simulink model "powerwindow05"  (Simulink 6.0)
settings: Solver=ode23t  StartTime=0.0  StopTime=inf  FixedStep=1e-4  RelTol=1e-2
InitFcn:
  | powericon('psbinitsys',bdroot);
values from neighbouring files (symbols this model uses):
  m = 50    [absdata.m]
libraries: powerlib x44, mblibv1 x18, simulink x8, dspquant2 x5, xpclib x4
(part 1 of 2)
settings Model: Creator=The MathWorks Inc.  LastModifiedBy=batserve  ExtModeAutoUpdateStatusClock=off
settings DataIOCC: SignalLoggingName=sigsOut
settings OptimizationCC: BooleanDataType=off
settings DebuggingCC: CheckExecutionContextPreStartOutputMsg=on  CheckExecutionContextRuntimeOutputMsg=on  SolverPrmCheckMsg=none  ParameterPrecisionLossMsg=none
settings HardwareCC: TargetUnknown=on
settings SimMechanicsCC: VisOnUpdateDiagram=on

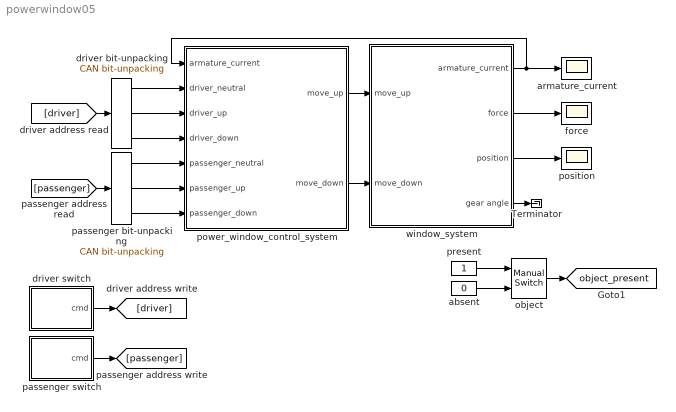
== system powerwindow05 ==
  Terminator : Terminator
  absent : Constant  Value=0
  armature_current : Scope
      settings: DataFormat=Array
  driver bit-unpacking : xpclib/CAN/Utilities/CAN bit-unpacking   bitpatterns={ [0:0] [1:1] [2:2] }  dtypes={ 'boolean' 'boolean' 'boolean' }
  driver switch : Subsystem  PropExecContextAcrossSSBoundary=on
  force : Scope
      settings: DataFormat=Array
  object : simulink/Signal Routing/Manual Switch  sw=1  action=0
  passenger bit-unpacking : xpclib/CAN/Utilities/CAN bit-unpacking   bitpatterns={ [0:0] [1:1] [2:2] }  dtypes={ 'boolean' 'boolean' 'boolean' }
  passenger switch : Subsystem  PropExecContextAcrossSSBoundary=on
  position : Scope
      settings: YMin=-0.05  YMax=0.5  DataFormat=Array
  power_window_control_system : Subsystem  PropExecContextAcrossSSBoundary=on
  present : Constant
  window_system : Subsystem  AncestorBlock=powerwindowlibphys/detailed_window_system  PropExecContextAcrossSSBoundary=on
  tag scope: object_present=global
  wires:
  power_window_control_system/1(move_up) -> window_system/1(move_up)
  power_window_control_system/2(move_down) -> window_system/2(move_down)
  window_system/1(armature_current) -> armature_current/1, power_window_control_system/1(armature_current)
  window_system/2(force) -> force/1
  window_system/3(position) -> position/1
  present/1 -> object/1
  absent/1 -> object/2
  object/1 -> [object_present]
  [passenger] -> passenger bit-unpacking/1
  [driver] -> driver bit-unpacking/1
  driver bit-unpacking/1 -> power_window_control_system/2(driver_neutral)
  driver bit-unpacking/2 -> power_window_control_system/3(driver_up)
  driver bit-unpacking/3 -> power_window_control_system/4(driver_down)
  passenger bit-unpacking/1 -> power_window_control_system/5(passenger_neutral)
  passenger bit-unpacking/2 -> power_window_control_system/6(passenger_up)
  passenger bit-unpacking/3 -> power_window_control_system/7(passenger_down)
  passenger switch/1(cmd) -> [passenger]
  driver switch/1(cmd) -> [driver]
  window_system/4(gear angle) -> Terminator/1

== system powerwindow05/driver switch ==
  CAN module : Subsystem  PropExecContextAcrossSSBoundary=on
  DAQ : Subsystem  PropExecContextAcrossSSBoundary=on
  GND : powerlib/Elements/Ground  Orientation=down  PhysicalDomain=powersysdomain  SubClassName=unknown  LeftPortType=p1  RightPortType=p1  LConnTagsString=a
  Vbattery 12[V] : powerlib/Electrical Sources/DC Voltage Source  Amplitude=12  Measurements=None
  control : Subsystem  PropExecContextAcrossSSBoundary=on
  switch : Subsystem  PropExecContextAcrossSSBoundary=on
  cmd : Outport
  wires:
  control/1(cmd) -> CAN module/1(command)
  CAN module/1(3bit) -> cmd/1
  DAQ/1(Out1) -> control/1(up)
  DAQ/2(Out2) -> control/2(down)
  connections:
  switch/RConn1 -- DAQ/LConn1
  switch/RConn2 -- DAQ/LConn2
  GND/LConn1 -- Vbattery 12[V]/LConn1
  Vbattery 12[V]/RConn1 -- switch/LConn1

== system powerwindow05/passenger switch ==
  CAN module : Subsystem  PropExecContextAcrossSSBoundary=on
  DAQ : Subsystem  PropExecContextAcrossSSBoundary=on
  GND : powerlib/Elements/Ground  Orientation=down  PhysicalDomain=powersysdomain  SubClassName=unknown  LeftPortType=p1  RightPortType=p1  LConnTagsString=a
  Vbattery 12[V] : powerlib/Electrical Sources/DC Voltage Source  Amplitude=12  Measurements=None
  control : Subsystem  PropExecContextAcrossSSBoundary=on
  switch : Subsystem  PropExecContextAcrossSSBoundary=on
  cmd : Outport
  wires:
  DAQ/2(Out2) -> control/2(down)
  DAQ/1(Out1) -> control/1(up)
  CAN module/1(3bit) -> cmd/1
  control/1(cmd) -> CAN module/1(command)
  connections:
  Vbattery 12[V]/RConn1 -- switch/LConn1
  GND/LConn1 -- Vbattery 12[V]/LConn1
  switch/RConn2 -- DAQ/LConn2
  switch/RConn1 -- DAQ/LConn1

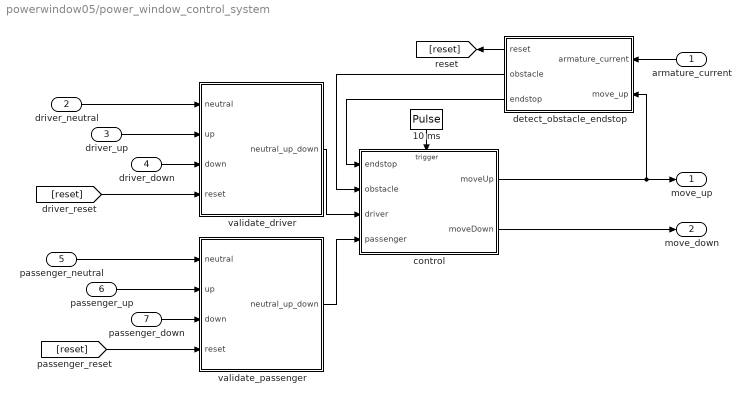
== system powerwindow05/power_window_control_system ==
  armature_current : Inport  Orientation=left  Port=1  LatchInput=off
  driver_neutral : Inport  Port=2  LatchInput=off
  driver_up : Inport  Port=3  LatchInput=off
  driver_down : Inport  Port=4  LatchInput=off
  passenger_neutral : Inport  Port=5  LatchInput=off
  passenger_up : Inport  Port=6  LatchInput=off
  passenger_down : Inport  Port=7  LatchInput=off
  10 ms : DiscretePulseGenerator  Orientation=down  SampleTime=10e-3
  control : Stateflow chart  TreatAsAtomicUnit=on  PropExecContextAcrossSSBoundary=on
  detect_obstacle_endstop : Subsystem  Orientation=left  PropExecContextAcrossSSBoundary=on
  validate_driver : Subsystem  PropExecContextAcrossSSBoundary=on
  validate_passenger : Subsystem  PropExecContextAcrossSSBoundary=on
  move_up : Outport
  move_down : Outport  Port=2
  wires:
  detect_obstacle_endstop/2(obstacle) -> control/2(obstacle)
  detect_obstacle_endstop/3(endstop) -> control/1(endstop)
  detect_obstacle_endstop/1(reset) -> [reset]
  armature_current/1 -> detect_obstacle_endstop/1(armature_current)
  10 ms/1 -> control/Trigger
  control/1(moveUp) -> detect_obstacle_endstop/2(move_up), move_up/1
  control/2(moveDown) -> move_down/1
  driver_neutral/1 -> validate_driver/1(neutral)
  driver_up/1 -> validate_driver/2(up)
  driver_down/1 -> validate_driver/3(down)
  [reset] -> validate_driver/4(reset)
  passenger_neutral/1 -> validate_passenger/1(neutral)
  passenger_up/1 -> validate_passenger/2(up)
  passenger_down/1 -> validate_passenger/3(down)
  [reset] -> validate_passenger/4(reset)
  validate_driver/1(neutral_up_down) -> control/3(driver)
  validate_passenger/1(neutral_up_down) -> control/4(passenger)

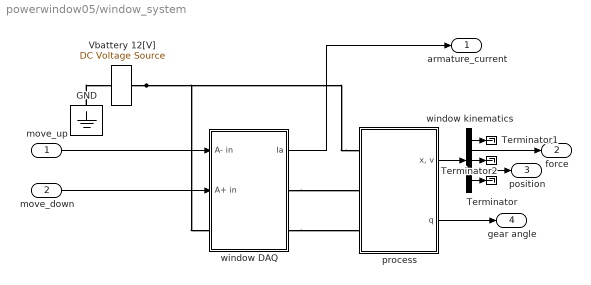
== system powerwindow05/window_system ==
  move_up : Inport  Port=1  LatchInput=off
  move_down : Inport  Port=2  LatchInput=off
  GND : powerlib/Elements/Ground  Orientation=down  PhysicalDomain=powersysdomain  SubClassName=unknown  LeftPortType=p1  RightPortType=p1  LConnTagsString=a
  Terminator : Terminator
  Terminator1 : Terminator
  Terminator2 : Terminator
  Vbattery 12[V] : powerlib/Electrical Sources/DC Voltage Source  Amplitude=12  Measurements=None
  process : Subsystem  AncestorBlock=powerwindowlibphys/process  PropExecContextAcrossSSBoundary=on
  window DAQ : Subsystem  PropExecContextAcrossSSBoundary=on
  window kinematics : Demux  Outputs=[1,1,2,1,4]
  armature_current : Outport
  force : Outport  Port=2
  position : Outport  Port=3
  gear angle : Outport  Port=4
  wires:
  process/2(q) -> gear angle/1
  process/1("x, v") -> window kinematics/1
  window DAQ/1(Ia) -> armature_current/1
  move_down/1 -> window DAQ/2(A+ in)
  move_up/1 -> window DAQ/1(A- in)
  window kinematics/3 -> Terminator2/1
  window kinematics/5 -> Terminator/1
  window kinematics/4 -> position/1
  window kinematics/1 -> Terminator1/1
  window kinematics/2 -> force/1
  connections:
  window DAQ/RConn2 -- process/LConn3
  window DAQ/RConn1 -- process/LConn2
  process/LConn1 -- window DAQ/LConn1 -- Vbattery 12[V]/RConn1
  GND/LConn1 -- Vbattery 12[V]/LConn1

== system powerwindow05/driver switch/CAN module ==
  command : Inport  Port=1  LatchInput=off
  "CAN bit-packing " : xpclib/CAN/Utilities/CAN bit-packing   bitpatterns={ [0:0] [1:1] [2:2]}
  Demux : Demux  Outputs=3
  3bit : Outport
  wires:
  "CAN bit-packing "/1 -> 3bit/1
  command/1 -> Demux/1
  Demux/1 -> "CAN bit-packing "/1
  Demux/2 -> "CAN bit-packing "/2
  Demux/3 -> "CAN bit-packing "/3

== system powerwindow05/driver switch/DAQ ==
  DAQ driver down : Subsystem  PropExecContextAcrossSSBoundary=on
  DAQ driver up : Subsystem  PropExecContextAcrossSSBoundary=on
  In1 : PMIOPort  Port=1  Side=Left
  In2 : PMIOPort  Port=2  Side=Left
  Out1 : Outport
  Out2 : Outport  Port=2
  wires:
  DAQ driver up/1(active) -> Out1/1
  DAQ driver down/1(active) -> Out2/1
  connections:
  In1/RConn1 -- DAQ driver up/LConn1
  In2/RConn1 -- DAQ driver down/LConn1

== system powerwindow05/driver switch/control ==
  up : Inport  Orientation=left  Port=1  LatchInput=off
  down : Inport  Orientation=left  Port=2  LatchInput=off
  Mux2 : Mux  Orientation=left  Inputs=2
  control input1 : DataTypeConversion  Orientation=left  OutDataTypeMode=boolean  SaturateOnIntegerOverflow=on  RndMeth=Zero
  control input2 : DataTypeConversion  Orientation=left  OutDataTypeMode=boolean  SaturateOnIntegerOverflow=on  RndMeth=Zero
  "driver neutral, up, down map" : CombinatorialLogic  Orientation=left  TruthTable=[1 0 0;0 0 1;0 1 0;1 0 0]
  cmd : Outport  Orientation=left
  wires:
  Mux2/1 -> "driver neutral, up, down map"/1
  control input1/1 -> Mux2/1
  control input2/1 -> Mux2/2
  up/1 -> control input1/1
  "driver neutral, up, down map"/1 -> cmd/1
  down/1 -> control input2/1

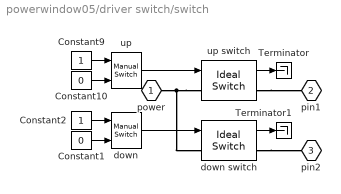
== system powerwindow05/driver switch/switch ==
  Constant1 : Constant  Value=0
  Constant10 : Constant  Value=0
  Constant2 : Constant
  Constant9 : Constant
  Terminator : Terminator
  Terminator1 : Terminator
  down : simulink/Signal Routing/Manual Switch  sw=0  action=0
  down switch : powerlib/Power Electronics/Ideal Switch  Ron=0.01  Lon=0  IC=0  Rs=1000000  Cs=inf  Measurements=on
  up : simulink/Signal Routing/Manual Switch  sw=0  action=0
  up switch : powerlib/Power Electronics/Ideal Switch  Ron=0.01  Lon=0  IC=0  Rs=1000000  Cs=inf  Measurements=on
  power : PMIOPort  Port=1  Side=Left
  pin1 : PMIOPort  Orientation=left  Port=2  Side=Right
  pin2 : PMIOPort  Orientation=left  Port=3  Side=Right
  wires:
  down/1 -> down switch/1
  down switch/1 -> Terminator1/1
  up/1 -> up switch/1
  up switch/1 -> Terminator/1
  Constant1/1 -> down/2
  Constant2/1 -> down/1
  Constant10/1 -> up/2
  Constant9/1 -> up/1
  connections:
  up switch/LConn1 -- power/RConn1 -- down switch/LConn1
  down switch/RConn1 -- pin2/RConn1
  up switch/RConn1 -- pin1/RConn1

== system powerwindow05/passenger switch/CAN module ==
  command : Inport  Port=1  LatchInput=off
  "CAN bit-packing " : xpclib/CAN/Utilities/CAN bit-packing   bitpatterns={ [0:0] [1:1] [2:2]}
  Demux : Demux  Outputs=3
  3bit : Outport
  wires:
  Demux/3 -> "CAN bit-packing "/3
  Demux/2 -> "CAN bit-packing "/2
  Demux/1 -> "CAN bit-packing "/1
  command/1 -> Demux/1
  "CAN bit-packing "/1 -> 3bit/1

== system powerwindow05/passenger switch/DAQ ==
  DAQ driver down : Subsystem  PropExecContextAcrossSSBoundary=on
  DAQ driver up : Subsystem  PropExecContextAcrossSSBoundary=on
  In1 : PMIOPort  Port=1  Side=Left
  In2 : PMIOPort  Port=2  Side=Left
  Out1 : Outport
  Out2 : Outport  Port=2
  wires:
  DAQ driver down/1(active) -> Out2/1
  DAQ driver up/1(active) -> Out1/1
  connections:
  In2/RConn1 -- DAQ driver down/LConn1
  In1/RConn1 -- DAQ driver up/LConn1

== system powerwindow05/passenger switch/control ==
  up : Inport  Orientation=left  Port=1  LatchInput=off
  down : Inport  Orientation=left  Port=2  LatchInput=off
  Mux2 : Mux  Orientation=left  Inputs=2
  control input1 : DataTypeConversion  Orientation=left  OutDataTypeMode=boolean  SaturateOnIntegerOverflow=on  RndMeth=Zero
  control input2 : DataTypeConversion  Orientation=left  OutDataTypeMode=boolean  SaturateOnIntegerOverflow=on  RndMeth=Zero
  "driver neutral, up, down map" : CombinatorialLogic  Orientation=left  TruthTable=[1 0 0;0 0 1;0 1 0;1 0 0]
  cmd : Outport  Orientation=left
  wires:
  down/1 -> control input2/1
  "driver neutral, up, down map"/1 -> cmd/1
  up/1 -> control input1/1
  control input2/1 -> Mux2/2
  control input1/1 -> Mux2/1
  Mux2/1 -> "driver neutral, up, down map"/1

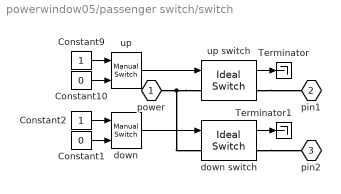
== system powerwindow05/passenger switch/switch ==
  Constant1 : Constant  Value=0
  Constant10 : Constant  Value=0
  Constant2 : Constant
  Constant9 : Constant
  Terminator : Terminator
  Terminator1 : Terminator
  down : simulink/Signal Routing/Manual Switch  sw=0  action=0
  down switch : powerlib/Power Electronics/Ideal Switch  Ron=0.01  Lon=0  IC=0  Rs=1000000  Cs=inf  Measurements=on
  up : simulink/Signal Routing/Manual Switch  sw=0  action=0
  up switch : powerlib/Power Electronics/Ideal Switch  Ron=0.01  Lon=0  IC=0  Rs=1000000  Cs=inf  Measurements=on
  power : PMIOPort  Port=1  Side=Left
  pin1 : PMIOPort  Orientation=left  Port=2  Side=Right
  pin2 : PMIOPort  Orientation=left  Port=3  Side=Right
  wires:
  Constant9/1 -> up/1
  Constant10/1 -> up/2
  Constant2/1 -> down/1
  Constant1/1 -> down/2
  up switch/1 -> Terminator/1
  up/1 -> up switch/1
  down switch/1 -> Terminator1/1
  down/1 -> down switch/1
  connections:
  up switch/RConn1 -- pin1/RConn1
  down switch/RConn1 -- pin2/RConn1
  up switch/LConn1 -- down switch/LConn1 -- power/RConn1

== system powerwindow05/power_window_control_system/detect_obstacle_endstop ==
  armature_current : Inport  Port=1  LatchInput=off
  move_up : Inport  Port=2  LatchInput=off
  detect_endstop : Subsystem  PropExecContextAcrossSSBoundary=on
  detect_obstacle : Subsystem  PropExecContextAcrossSSBoundary=on
  either : Logic  Operator=OR
  process_current : Subsystem  PropExecContextAcrossSSBoundary=on
  reset : Outport
  obstacle : Outport  Port=2
  endstop : Outport  Port=3
  wires:
  process_current/1(processed_current) -> detect_endstop/1(armature_current), detect_obstacle/2(armature_current)
  move_up/1 -> detect_obstacle/1(move_up)
  either/1 -> reset/1
  detect_endstop/1(endstop) -> either/2, endstop/1
  detect_obstacle/1(obstacle) -> obstacle/1, either/1
  armature_current/1 -> process_current/1(raw_current)

== system powerwindow05/power_window_control_system/validate_driver ==
  neutral : Inport  Port=1  LatchInput=off
  up : Inport  Port=2  LatchInput=off
  down : Inport  Port=3  LatchInput=off
  reset : Inport  Port=4  LatchInput=off
  Mux : Mux  Inputs=3
  check_down : Subsystem  PropExecContextAcrossSSBoundary=on
  check_up : Subsystem  PropExecContextAcrossSSBoundary=on
  mutually_exclusive : Subsystem  PropExecContextAcrossSSBoundary=on
  neutral_up_down : Outport
  wires:
  Mux/1 -> neutral_up_down/1
  reset/1 -> [reset]
  [reset] -> check_down/2(reset)
  [reset] -> check_up/2(reset)
  check_up/1(checked_action) -> mutually_exclusive/2(up)
  neutral/1 -> mutually_exclusive/1(neutral)
  up/1 -> check_up/1(action)
  down/1 -> check_down/1(action)
  mutually_exclusive/1(validated_neutral) -> Mux/1
  mutually_exclusive/2(validated_up) -> Mux/2
  mutually_exclusive/3(validated_down) -> Mux/3
  check_down/1(checked_action) -> mutually_exclusive/3(down)

== system powerwindow05/power_window_control_system/validate_passenger ==
  neutral : Inport  Port=1  LatchInput=off
  up : Inport  Port=2  LatchInput=off
  down : Inport  Port=3  LatchInput=off
  reset : Inport  Port=4  LatchInput=off
  Mux : Mux  Inputs=3
  check_down : Subsystem  PropExecContextAcrossSSBoundary=on
  check_up : Subsystem  PropExecContextAcrossSSBoundary=on
  mutually_exclusive : Subsystem  PropExecContextAcrossSSBoundary=on
  neutral_up_down : Outport
  wires:
  Mux/1 -> neutral_up_down/1
  reset/1 -> [reset]
  [reset] -> check_down/2(reset)
  [reset] -> check_up/2(reset)
  check_up/1(checked_action) -> mutually_exclusive/2(up)
  neutral/1 -> mutually_exclusive/1(neutral)
  up/1 -> check_up/1(action)
  down/1 -> check_down/1(action)
  mutually_exclusive/1(validated_neutral) -> Mux/1
  mutually_exclusive/2(validated_up) -> Mux/2
  mutually_exclusive/3(validated_down) -> Mux/3
  check_down/1(checked_action) -> mutually_exclusive/3(down)

== system powerwindow05/window_system/process ==
  actuator : Subsystem  PropExecContextAcrossSSBoundary=on
  ideal Ia : Scope
      settings: YMin=-7.5  YMax=20  SaveName=ScopeData4
  plant : Subsystem  PropExecContextAcrossSSBoundary=on
  Vcc : PMIOPort  Port=1  Side=Left
  A- : PMIOPort  Port=2  Side=Left
  A+ : PMIOPort  Port=3  Side=Left
  "x, v" : Outport
  q : Outport  Port=2
  wires:
  plant/3(q) -> q/1
  plant/2("F, x, v") -> "x, v"/1
  actuator/2(wL) -> plant/1(wi)
  actuator/1(Ia) -> ideal Ia/1
  plant/1(ti) -> actuator/1(tL)
  connections:
  A+/RConn1 -- actuator/LConn3
  A-/RConn1 -- actuator/LConn2
  Vcc/RConn1 -- actuator/LConn1

== system powerwindow05/window_system/window DAQ ==
  A- in : Inport  Port=1  LatchInput=off
  A+ in : Inport  Port=2  LatchInput=off
  ADC Ia : Subsystem  PropExecContextAcrossSSBoundary=on  mask(AD Converter){Ts=0.01, peak=3.5, Td=0.005, bits=8}
      mask prompts: Ts "sample time (-1 for inherited)"; Td "delay (-1 for inherited)"
      mask help: Analog (A) to digital (D) converter with sample rate, conversion delay, range, and number of bits used for conversion.
      mask Display:
      | plot([0.5 1.5 1.5 2.5 2.5 3.5 3.5 4.5], [0 0 1 1 2 2 3 3])
      | plot([0 3], [0 3])
  DAC down : ZeroOrderHold  SampleTime=0.01
  DAC up : ZeroOrderHold  SampleTime=0.01
  amplification down : Subsystem  PropExecContextAcrossSSBoundary=on
  amplification up : Subsystem  PropExecContextAcrossSSBoundary=on
  conditioning Ia measurement : Subsystem  PropExecContextAcrossSSBoundary=on
  Vcc : PMIOPort  Port=1  Side=Left
  A- out : PMIOPort  Orientation=left  Port=2  Side=Right
  A+ out : PMIOPort  Orientation=left  Port=3  Side=Right
  Ia : Outport
  wires:
  A+ in/1 -> DAC down/1
  A- in/1 -> DAC up/1
  ADC Ia/1(D) -> Ia/1
  conditioning Ia measurement/1(Vmeas) -> ADC Ia/1(A)
  DAC down/1 -> amplification down/1(on)
  DAC up/1 -> amplification up/1(on)
  connections:
  amplification down/RConn1 -- A+ out/RConn1
  conditioning Ia measurement/RConn1 -- A- out/RConn1
  amplification up/RConn1 -- conditioning Ia measurement/LConn1
  Vcc/RConn1 -- amplification down/LConn1 -- amplification up/LConn1

== system powerwindow05/driver switch/DAQ/DAQ driver down ==
  ADC driver up : Subsystem  Orientation=left  PropExecContextAcrossSSBoundary=on  mask(AD Converter){Ts=0.01, Td=0.005, peak=4.9, bits=2}
      mask prompts: Ts "sample time (-1 for inherited)"; Td "delay (-1 for inherited)"
      mask help: Analog (A) to digital (D) converter with sample rate, conversion delay, range, and number of bits used for conversion.
      mask init:
      | gain = peak / (2^(bits-1));
      mask Display:
      | plot([0.5 1.5 1.5 2.5 2.5 3.5 3.5 4.5], [0 0 1 1 2 2 3 3])
      | plot([0 3], [0 3])
  conditioning driver up : Subsystem  Orientation=left  PropExecContextAcrossSSBoundary=on
  Vin : PMIOPort  Orientation=left  Port=1  Side=Left
  active : Outport  Orientation=left
  wires:
  ADC driver up/1(D) -> active/1
  conditioning driver up/1(active) -> ADC driver up/1(A)
  connections:
  Vin/RConn1 -- conditioning driver up/LConn1

== system powerwindow05/driver switch/DAQ/DAQ driver up ==
  ADC driver up : Subsystem  Orientation=left  PropExecContextAcrossSSBoundary=on  mask(AD Converter){Ts=0.01, Td=0.005, peak=4.9, bits=2}
      mask prompts: Ts "sample time (-1 for inherited)"; Td "delay (-1 for inherited)"
      mask help: Analog (A) to digital (D) converter with sample rate, conversion delay, range, and number of bits used for conversion.
      mask init:
      | gain = peak / (2^(bits-1));
      mask Display:
      | plot([0.5 1.5 1.5 2.5 2.5 3.5 3.5 4.5], [0 0 1 1 2 2 3 3])
      | plot([0 3], [0 3])
  conditioning driver up : Subsystem  Orientation=left  PropExecContextAcrossSSBoundary=on
  Vin : PMIOPort  Orientation=left  Port=1  Side=Left
  active : Outport  Orientation=left
  wires:
  conditioning driver up/1(active) -> ADC driver up/1(A)
  ADC driver up/1(D) -> active/1
  connections:
  Vin/RConn1 -- conditioning driver up/LConn1

== system powerwindow05/passenger switch/DAQ/DAQ driver down ==
  ADC driver up : Subsystem  Orientation=left  PropExecContextAcrossSSBoundary=on  mask(AD Converter){Ts=0.01, Td=0.005, peak=4.9, bits=2}
      mask prompts: Ts "sample time (-1 for inherited)"; Td "delay (-1 for inherited)"
      mask help: Analog (A) to digital (D) converter with sample rate, conversion delay, range, and number of bits used for conversion.
      mask init:
      | gain = peak / (2^(bits-1));
      mask Display:
      | plot([0.5 1.5 1.5 2.5 2.5 3.5 3.5 4.5], [0 0 1 1 2 2 3 3])
      | plot([0 3], [0 3])
  conditioning driver up : Subsystem  Orientation=left  PropExecContextAcrossSSBoundary=on
  Vin : PMIOPort  Orientation=left  Port=1  Side=Left
  active : Outport  Orientation=left
  wires:
  conditioning driver up/1(active) -> ADC driver up/1(A)
  ADC driver up/1(D) -> active/1
  connections:
  Vin/RConn1 -- conditioning driver up/LConn1

== system powerwindow05/passenger switch/DAQ/DAQ driver up ==
  ADC driver up : Subsystem  Orientation=left  PropExecContextAcrossSSBoundary=on  mask(AD Converter){Ts=0.01, Td=0.005, peak=4.9, bits=2}
      mask prompts: Ts "sample time (-1 for inherited)"; Td "delay (-1 for inherited)"
      mask help: Analog (A) to digital (D) converter with sample rate, conversion delay, range, and number of bits used for conversion.
      mask init:
      | gain = peak / (2^(bits-1));
      mask Display:
      | plot([0.5 1.5 1.5 2.5 2.5 3.5 3.5 4.5], [0 0 1 1 2 2 3 3])
      | plot([0 3], [0 3])
  conditioning driver up : Subsystem  Orientation=left  PropExecContextAcrossSSBoundary=on
  Vin : PMIOPort  Orientation=left  Port=1  Side=Left
  active : Outport  Orientation=left
  wires:
  ADC driver up/1(D) -> active/1
  conditioning driver up/1(active) -> ADC driver up/1(A)
  connections:
  Vin/RConn1 -- conditioning driver up/LConn1

== system powerwindow05/power_window_control_system/detect_obstacle_endstop/detect_endstop ==
  armature_current : Inport  Port=1  LatchInput=off
  current_limit : simulink/Logic and Bit Operations/Compare To Constant  relop=>  const=15  LogicOutDataTypeMode=uint8
  passenger control : DataTypeConversion  OutDataTypeMode=boolean  SaturateOnIntegerOverflow=on  RndMeth=Zero
  endstop : Outport
  wires:
  armature_current/1 -> current_limit/1
  current_limit/1 -> passenger control/1
  passenger control/1 -> endstop/1

== system powerwindow05/power_window_control_system/detect_obstacle_endstop/detect_obstacle ==
  move_up : Inport  Orientation=left  Port=1  LatchInput=off
  armature_current : Inport  Port=2  LatchInput=off
  10 ms : DiscretePulseGenerator  Orientation=down  SampleTime=10e-3
  Multiply : Product  Orientation=up  Inputs=**  OutDataType=sfix(8)  OutScaling=2^-5
  break dependency : UnitDelay  Orientation=left  SampleTime=0.01
  current_limit : simulink/Logic and Bit Operations/Compare To Constant  relop=>  const=1.1  LogicOutDataTypeMode=uint8
  delay_detection : Stateflow chart  Orientation=left  TreatAsAtomicUnit=on  PropExecContextAcrossSSBoundary=on
  passenger control : DataTypeConversion  Orientation=up  OutDataTypeMode=boolean  SaturateOnIntegerOverflow=on  RndMeth=Zero
  obstacle : Outport  Orientation=up
  wires:
  current_limit/1 -> Multiply/1
  delay_detection/1(detect) -> Multiply/2
  armature_current/1 -> current_limit/1
  move_up/1 -> break dependency/1
  Multiply/1 -> passenger control/1
  10 ms/1 -> delay_detection/Trigger
  break dependency/1 -> delay_detection/1(move_up)
  passenger control/1 -> obstacle/1

== system powerwindow05/power_window_control_system/detect_obstacle_endstop/process_current ==
  raw_current : Inport  Port=1  LatchInput=off
  3.5 / (2^(bits-1)) : Gain  Gain=0.02734375  ParameterDataType=sfix( 8 )  ParameterScaling=2^-12  OutDataTypeMode=Specify via dialog  OutScaling=2^-6
  Abs : Abs
  gain : Gain  Gain=5  ParameterDataType=sfix( 8 )  ParameterScaling=2^-4  OutDataTypeMode=Specify via dialog  OutScaling=2^-5
  processed_current : Outport
  wires:
  3.5 / (2^(bits-1))/1 -> gain/1
  gain/1 -> Abs/1
  Abs/1 -> processed_current/1
  raw_current/1 -> 3.5 / (2^(bits-1))/1

== system powerwindow05/power_window_control_system/validate_driver/check_down ==
  action : Inport  Port=1  LatchInput=off
  reset : Inport  Port=2  LatchInput=off
  allow_action : Logic
  overrule : Logic  Operator=NOT
  checked_action : Outport
  wires:
  reset/1 -> overrule/1
  allow_action/1 -> checked_action/1
  action/1 -> allow_action/1
  overrule/1 -> allow_action/2

== system powerwindow05/power_window_control_system/validate_driver/check_up ==
  action : Inport  Port=1  LatchInput=off
  reset : Inport  Port=2  LatchInput=off
  allow_action : Logic
  overrule : Logic  Operator=NOT
  checked_action : Outport
  wires:
  overrule/1 -> allow_action/2
  action/1 -> allow_action/1
  allow_action/1 -> checked_action/1
  reset/1 -> overrule/1

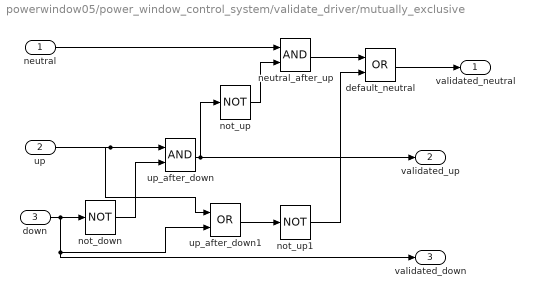
== system powerwindow05/power_window_control_system/validate_driver/mutually_exclusive ==
  neutral : Inport  Port=1  LatchInput=off
  up : Inport  Port=2  LatchInput=off
  down : Inport  Port=3  LatchInput=off
  default_neutral : Logic  Operator=OR
  neutral_after_up : Logic
  not_down : Logic  Operator=NOT
  not_up : Logic  Operator=NOT
  not_up1 : Logic  Operator=NOT
  up_after_down : Logic
  up_after_down1 : Logic  Operator=OR
  validated_neutral : Outport
  validated_up : Outport  Port=2
  validated_down : Outport  Port=3
  wires:
  not_down/1 -> up_after_down/2
  up_after_down/1 -> not_up/1, validated_up/1
  not_up/1 -> neutral_after_up/2
  down/1 -> not_down/1, up_after_down1/2, validated_down/1
  neutral/1 -> neutral_after_up/1
  up/1 -> up_after_down/1, up_after_down1/1
  up_after_down1/1 -> not_up1/1
  neutral_after_up/1 -> default_neutral/1
  default_neutral/1 -> validated_neutral/1
  not_up1/1 -> default_neutral/2

== system powerwindow05/power_window_control_system/validate_passenger/check_down ==
  action : Inport  Port=1  LatchInput=off
  reset : Inport  Port=2  LatchInput=off
  allow_action : Logic
  overrule : Logic  Operator=NOT
  checked_action : Outport
  wires:
  reset/1 -> overrule/1
  allow_action/1 -> checked_action/1
  action/1 -> allow_action/1
  overrule/1 -> allow_action/2

== system powerwindow05/power_window_control_system/validate_passenger/check_up ==
  action : Inport  Port=1  LatchInput=off
  reset : Inport  Port=2  LatchInput=off
  allow_action : Logic
  overrule : Logic  Operator=NOT
  checked_action : Outport
  wires:
  overrule/1 -> allow_action/2
  action/1 -> allow_action/1
  allow_action/1 -> checked_action/1
  reset/1 -> overrule/1

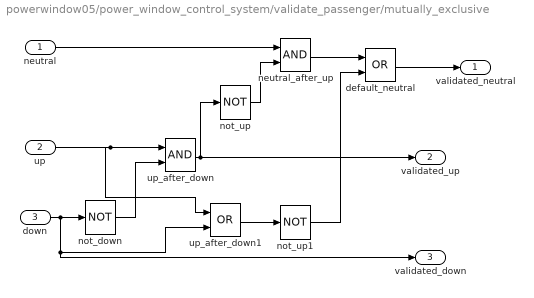
== system powerwindow05/power_window_control_system/validate_passenger/mutually_exclusive ==
  neutral : Inport  Port=1  LatchInput=off
  up : Inport  Port=2  LatchInput=off
  down : Inport  Port=3  LatchInput=off
  default_neutral : Logic  Operator=OR
  neutral_after_up : Logic
  not_down : Logic  Operator=NOT
  not_up : Logic  Operator=NOT
  not_up1 : Logic  Operator=NOT
  up_after_down : Logic
  up_after_down1 : Logic  Operator=OR
  validated_neutral : Outport
  validated_up : Outport  Port=2
  validated_down : Outport  Port=3
  wires:
  not_down/1 -> up_after_down/2
  up_after_down/1 -> not_up/1, validated_up/1
  not_up/1 -> neutral_after_up/2
  down/1 -> not_down/1, up_after_down1/2, validated_down/1
  neutral/1 -> neutral_after_up/1
  up/1 -> up_after_down/1, up_after_down1/1
  up_after_down1/1 -> not_up1/1
  neutral_after_up/1 -> default_neutral/1
  default_neutral/1 -> validated_neutral/1
  not_up1/1 -> default_neutral/2

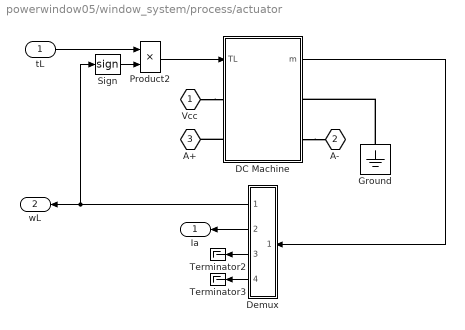
== system powerwindow05/window_system/process/actuator ==
  tL : Inport  Port=1  LatchInput=off
  DC Machine : Subsystem  PropExecContextAcrossSSBoundary=on  mask(DC machine){RLa=[0.15  0.036], RLf=[1.5 3], Laf=1, J=0.085, Bm=5, Tf=0, w0=0, PSBOutputType=110}
      mask prompts: RLa "Armature resistance and inductance [Ra (ohms) La (H) ]"; RLf "Field resistance and inductance [Rf (ohms) Lf (H) ]"; Laf "Field-armature mutual inductance Laf (H) :"; J "Total inertia J (kg.m^2)"; Bm "Viscous friction coefficient Bm (N.m.s)"; Tf "Coulomb friction torque Tf (N.m)"; w0 "Initial speed (rad/s) :"; PSBOutputType "Output type"
      mask help:
      | This block implements a separately excited DC machine. Access is provided  to the field connections so that the machine can be used as a shunt-connected or a series-connected  DC machine.
      |
      | Input 1 and output 1 : positive and negative armature terminals
      | Input 2 and output 2 : positive and negative field terminals
      | Input 3    : Load torque
      | Output 3 : Simulink measurement output [ w Ia If Te ]
      mask init:
      | Ra=RLa(1); La=RLa(2);
      | Rf=RLf(1); Lf=RLf(2);
      mask Help: web(psbhelp)
      mask Display: plot(-80,-80,80,80,[0,9,18,24,29,30,29,24,18,9,0,-9,-18,-24,-29,-30,-29,-24,-18,-9,0],[30,29,24,18,9,0,-9,-18,-24,-29,-30,-29,-24,-18,-9,0,9,18,24,29,30],[-29,-35,-35,-29],[-8,-8,8,8],[29,35,35,29],[-8,-8,8,8],[-35,-55],[0,0],[35,55],[0,0],[-78,-50,-50,-49,-45,-39,-33,-26,-21,-18,-17,-19,-22,-22,-26,-27,-25,-22,-16,-9,-3,2,6,6,4,1,1,-3,-4,-2,2,7,14,20,26,29,30,28,24,24,21,20,21,25,31,37,44,49,50,50,50,78]*.7,[58,58,57.2,49.2,42.8,38.8,38,39.6,44.4,51.6,59.6,67.6,72.4,72.4,65.2,57.2,49.2,42.8,38.8,38,39.6,44.4,51.6,59.6,67.6,72.4,72.4,65.2,57.2,49.2,42.8,38.8,38,39.6,44.4,51.6,59.6,67.6,72.4,72.4,65.2,57.2,49.2,42.8,38.8,38,39.6,44.4,51.6,58,58,58]*.6+15 );
  Demux : Subsystem  Orientation=left  PropExecContextAcrossSSBoundary=on
  Ground : powerlib/Elements/Ground  Orientation=down  PhysicalDomain=powersysdomain  SubClassName=unknown  LeftPortType=p1  RightPortType=p1  LConnTagsString=a
  Product2 : Product  SaturateOnIntegerOverflow=on  InputSameDT=on
  Sign : Signum
  Terminator2 : Terminator
  Terminator3 : Terminator
  Vcc : PMIOPort  Port=1  Side=Left
  A- : PMIOPort  Orientation=left  Port=2  Side=Left
  A+ : PMIOPort  Port=3  Side=Left
  Ia : Outport  Orientation=left
  wL : Outport  Orientation=left  Port=2
  wires:
  Product2/1 -> DC Machine/1(TL)
  Demux/1(wm) -> Sign/1, wL/1
  Demux/2(Ia) -> Ia/1
  tL/1 -> Product2/1
  Sign/1 -> Product2/2
  DC Machine/1(m) -> Demux/1(m)
  Demux/3(If) -> Terminator2/1
  Demux/4(Te) -> Terminator3/1
  connections:
  DC Machine/RConn2 -- A-/RConn1
  Ground/LConn1 -- DC Machine/RConn1
  DC Machine/LConn2 -- A+/RConn1
  Vcc/RConn1 -- DC Machine/LConn1

== system powerwindow05/window_system/process/plant ==
  wi : Inport  Port=1  LatchInput=off
  Demux1 : Demux  Outputs=[4, 1, 2, 1, 1]
  Terminator : Terminator
  Terminator1 : Terminator
  Terminator2 : Terminator
  object : Subsystem  PropExecContextAcrossSSBoundary=on
  window : Subsystem  PropExecContextAcrossSSBoundary=on
  ti : Outport
  "F, x, v" : Outport  Port=2
  q : Outport  Port=3
  wires:
  window/1(ti) -> ti/1
  wi/1 -> window/1(wi)
  object/1(torque) -> window/2(Fx)
  window/3(q) -> q/1
  Demux1/4 -> object/2(velocity)
  Demux1/2 -> object/1(position)
  Demux1/1 -> Terminator/1
  Demux1/3 -> Terminator1/1
  Demux1/5 -> Terminator2/1
  window/2(F,d,v) -> Demux1/1, "F, x, v"/1

== system powerwindow05/window_system/window DAQ/ADC Ia ==
  A : Inport  Port=1  LatchInput=off
  Uniform Encoder : dspquant2/Uniform Encoder  peak=peak  bits=bits  otype=Signed integer
  Unit Delay : UnitDelay  SampleTime=Td
  Zero-Order Hold : ZeroOrderHold  SampleTime=Ts
  D : Outport
  wires:
  Zero-Order Hold/1 -> Uniform Encoder/1
  Unit Delay/1 -> Zero-Order Hold/1
  A/1 -> Unit Delay/1
  Uniform Encoder/1 -> D/1

== system powerwindow05/window_system/window DAQ/amplification down ==
  on : Inport  Port=1  LatchInput=off
  Logical Operator : Logic  Operator=NOT
  Terminator1 : Terminator
  Terminator2 : Terminator
  high switch : powerlib/Power Electronics/Ideal Switch  Ron=0.01  Lon=0  IC=0  Rs=1000000  Cs=inf  Measurements=on
  low switch : powerlib/Power Electronics/Ideal Switch  Ron=0.01  Lon=0  IC=0  Rs=1000000  Cs=inf  Measurements=on
  output Ground1 : powerlib/Elements/Ground  Orientation=down  PhysicalDomain=powersysdomain  SubClassName=unknown  LeftPortType=p1  RightPortType=p1  LConnTagsString=a
  Vcc : PMIOPort  Port=1  Side=Left
  pin1 : PMIOPort  Orientation=left  Port=2  Side=Right
  wires:
  Logical Operator/1 -> low switch/1
  high switch/1 -> Terminator1/1
  on/1 -> high switch/1, Logical Operator/1
  low switch/1 -> Terminator2/1
  connections:
  pin1/RConn1 -- high switch/RConn1 -- low switch/RConn1
  output Ground1/LConn1 -- low switch/LConn1
  high switch/LConn1 -- Vcc/RConn1

== system powerwindow05/window_system/window DAQ/amplification up ==
  on : Inport  Port=1  LatchInput=off
  Logical Operator : Logic  Operator=NOT
  Terminator1 : Terminator
  Terminator2 : Terminator
  high switch : powerlib/Power Electronics/Ideal Switch  Ron=0.01  Lon=0  IC=0  Rs=1000000  Cs=inf  Measurements=on
  low switch : powerlib/Power Electronics/Ideal Switch  Ron=0.01  Lon=0  IC=0  Rs=1000000  Cs=inf  Measurements=on
  output Ground1 : powerlib/Elements/Ground  Orientation=down  PhysicalDomain=powersysdomain  SubClassName=unknown  LeftPortType=p1  RightPortType=p1  LConnTagsString=a
  Vcc : PMIOPort  Port=1  Side=Left
  pin1 : PMIOPort  Orientation=left  Port=2  Side=Right
  wires:
  Logical Operator/1 -> low switch/1
  high switch/1 -> Terminator1/1
  on/1 -> Logical Operator/1, high switch/1
  low switch/1 -> Terminator2/1
  connections:
  output Ground1/LConn1 -- low switch/LConn1
  high switch/LConn1 -- Vcc/RConn1
  pin1/RConn1 -- low switch/RConn1 -- high switch/RConn1

== system powerwindow05/window_system/window DAQ/conditioning Ia measurement ==
  R1 : powerlib/Elements/Series RLC Branch  PhysicalDomain=powersysdomain  SubClassName=unknown  LeftPortType=p1  RightPortType=p1  LConnTagsString=__new0  RConnTagsString=__new0  Resistance=0.18  Inductance=0  Capacitance=inf  Measurements=None
  measure1 : powerlib/Measurements/Voltage Measurement  Orientation=up  PhasorSimulation=off  OutputType=Magnitude  PSBequivalent=0
  Vin : PMIOPort  Port=1  Side=Left
  Vout : PMIOPort  Orientation=left  Port=2  Side=Right
  Vmeas : Outport  Orientation=up
  wires:
  measure1/1 -> Vmeas/1
  connections:
  Vin/RConn1 -- measure1/LConn1 -- R1/LConn1
  R1/RConn1 -- Vout/RConn1 -- measure1/LConn2

== system powerwindow05/driver switch/DAQ/DAQ driver down/ADC driver up ==
  A : Inport  Port=1  LatchInput=off
  Gain : Gain  Gain=gain  SaturateOnIntegerOverflow=on
  Uniform Encoder : dspquant2/Uniform Encoder  peak=peak  bits=bits  otype=Signed integer
  Unit Delay : UnitDelay  SampleTime=Td
  Zero-Order Hold : ZeroOrderHold  SampleTime=Ts
  type : DataTypeConversion  OutDataTypeMode=double  SaturateOnIntegerOverflow=on  RndMeth=Zero
  D : Outport
  wires:
  Zero-Order Hold/1 -> Uniform Encoder/1
  Unit Delay/1 -> Zero-Order Hold/1
  A/1 -> Unit Delay/1
  Uniform Encoder/1 -> type/1
  type/1 -> Gain/1
  Gain/1 -> D/1

== system powerwindow05/driver switch/DAQ/DAQ driver down/conditioning driver up ==
  R1 : powerlib/Elements/Series RLC Branch  PhysicalDomain=powersysdomain  SubClassName=unknown  LeftPortType=p1  RightPortType=p1  LConnTagsString=__new0  RConnTagsString=__new0  Resistance=6800  Inductance=0  Capacitance=inf  Measurements=None
  R2 : powerlib/Elements/Series RLC Branch  Orientation=up  PhysicalDomain=powersysdomain  SubClassName=unknown  LeftPortType=p1  RightPortType=p1  LConnTagsString=__new0  RConnTagsString=__new0  Resistance=4700  Inductance=0  Capacitance=inf  Measurements=None
  measure1 : powerlib/Measurements/Voltage Measurement  PhasorSimulation=off  OutputType=Magnitude  PSBequivalent=0
  output Ground2 : powerlib/Elements/Ground  Orientation=down  PhysicalDomain=powersysdomain  SubClassName=unknown  LeftPortType=p1  RightPortType=p1  LConnTagsString=a
  output Ground3 : powerlib/Elements/Ground  Orientation=down  PhysicalDomain=powersysdomain  SubClassName=unknown  LeftPortType=p1  RightPortType=p1  LConnTagsString=a
  Vin : PMIOPort  Port=1  Side=Left
  active : Outport
  wires:
  measure1/1 -> active/1
  connections:
  output Ground3/LConn1 -- measure1/LConn2
  output Ground2/LConn1 -- R2/LConn1
  Vin/RConn1 -- R1/LConn1
  measure1/LConn1 -- R2/RConn1 -- R1/RConn1

== system powerwindow05/driver switch/DAQ/DAQ driver up/ADC driver up ==
  A : Inport  Port=1  LatchInput=off
  Gain : Gain  Gain=gain  SaturateOnIntegerOverflow=on
  Uniform Encoder : dspquant2/Uniform Encoder  peak=peak  bits=bits  otype=Signed integer
  Unit Delay : UnitDelay  SampleTime=Td
  Zero-Order Hold : ZeroOrderHold  SampleTime=Ts
  type : DataTypeConversion  OutDataTypeMode=double  SaturateOnIntegerOverflow=on  RndMeth=Zero
  D : Outport
  wires:
  Gain/1 -> D/1
  type/1 -> Gain/1
  Uniform Encoder/1 -> type/1
  A/1 -> Unit Delay/1
  Unit Delay/1 -> Zero-Order Hold/1
  Zero-Order Hold/1 -> Uniform Encoder/1

== system powerwindow05/driver switch/DAQ/DAQ driver up/conditioning driver up ==
  R1 : powerlib/Elements/Series RLC Branch  PhysicalDomain=powersysdomain  SubClassName=unknown  LeftPortType=p1  RightPortType=p1  LConnTagsString=__new0  RConnTagsString=__new0  Resistance=6800  Inductance=0  Capacitance=inf  Measurements=None
  R2 : powerlib/Elements/Series RLC Branch  Orientation=up  PhysicalDomain=powersysdomain  SubClassName=unknown  LeftPortType=p1  RightPortType=p1  LConnTagsString=__new0  RConnTagsString=__new0  Resistance=4700  Inductance=0  Capacitance=inf  Measurements=None
  measure1 : powerlib/Measurements/Voltage Measurement  PhasorSimulation=off  OutputType=Magnitude  PSBequivalent=0
  output Ground2 : powerlib/Elements/Ground  Orientation=down  PhysicalDomain=powersysdomain  SubClassName=unknown  LeftPortType=p1  RightPortType=p1  LConnTagsString=a
  output Ground3 : powerlib/Elements/Ground  Orientation=down  PhysicalDomain=powersysdomain  SubClassName=unknown  LeftPortType=p1  RightPortType=p1  LConnTagsString=a
  Vin : PMIOPort  Port=1  Side=Left
  active : Outport
  wires:
  measure1/1 -> active/1
  connections:
  measure1/LConn1 -- R1/RConn1 -- R2/RConn1
  Vin/RConn1 -- R1/LConn1
  output Ground2/LConn1 -- R2/LConn1
  output Ground3/LConn1 -- measure1/LConn2

== system powerwindow05/passenger switch/DAQ/DAQ driver down/ADC driver up ==
  A : Inport  Port=1  LatchInput=off
  Gain : Gain  Gain=gain  SaturateOnIntegerOverflow=on
  Uniform Encoder : dspquant2/Uniform Encoder  peak=peak  bits=bits  otype=Signed integer
  Unit Delay : UnitDelay  SampleTime=Td
  Zero-Order Hold : ZeroOrderHold  SampleTime=Ts
  type : DataTypeConversion  OutDataTypeMode=double  SaturateOnIntegerOverflow=on  RndMeth=Zero
  D : Outport
  wires:
  Gain/1 -> D/1
  type/1 -> Gain/1
  Uniform Encoder/1 -> type/1
  A/1 -> Unit Delay/1
  Unit Delay/1 -> Zero-Order Hold/1
  Zero-Order Hold/1 -> Uniform Encoder/1

== system powerwindow05/passenger switch/DAQ/DAQ driver down/conditioning driver up ==
  R1 : powerlib/Elements/Series RLC Branch  PhysicalDomain=powersysdomain  SubClassName=unknown  LeftPortType=p1  RightPortType=p1  LConnTagsString=__new0  RConnTagsString=__new0  Resistance=6800  Inductance=0  Capacitance=inf  Measurements=None
  R2 : powerlib/Elements/Series RLC Branch  Orientation=up  PhysicalDomain=powersysdomain  SubClassName=unknown  LeftPortType=p1  RightPortType=p1  LConnTagsString=__new0  RConnTagsString=__new0  Resistance=4700  Inductance=0  Capacitance=inf  Measurements=None
  measure1 : powerlib/Measurements/Voltage Measurement  PhasorSimulation=off  OutputType=Magnitude  PSBequivalent=0
  output Ground2 : powerlib/Elements/Ground  Orientation=down  PhysicalDomain=powersysdomain  SubClassName=unknown  LeftPortType=p1  RightPortType=p1  LConnTagsString=a
  output Ground3 : powerlib/Elements/Ground  Orientation=down  PhysicalDomain=powersysdomain  SubClassName=unknown  LeftPortType=p1  RightPortType=p1  LConnTagsString=a
  Vin : PMIOPort  Port=1  Side=Left
  active : Outport
  wires:
  measure1/1 -> active/1
  connections:
  R1/RConn1 -- R2/RConn1 -- measure1/LConn1
  Vin/RConn1 -- R1/LConn1
  output Ground2/LConn1 -- R2/LConn1
  output Ground3/LConn1 -- measure1/LConn2

== system powerwindow05/passenger switch/DAQ/DAQ driver up/ADC driver up ==
  A : Inport  Port=1  LatchInput=off
  Gain : Gain  Gain=gain  SaturateOnIntegerOverflow=on
  Uniform Encoder : dspquant2/Uniform Encoder  peak=peak  bits=bits  otype=Signed integer
  Unit Delay : UnitDelay  SampleTime=Td
  Zero-Order Hold : ZeroOrderHold  SampleTime=Ts
  type : DataTypeConversion  OutDataTypeMode=double  SaturateOnIntegerOverflow=on  RndMeth=Zero
  D : Outport
  wires:
  Zero-Order Hold/1 -> Uniform Encoder/1
  Unit Delay/1 -> Zero-Order Hold/1
  A/1 -> Unit Delay/1
  Uniform Encoder/1 -> type/1
  type/1 -> Gain/1
  Gain/1 -> D/1

== system powerwindow05/passenger switch/DAQ/DAQ driver up/conditioning driver up ==
  R1 : powerlib/Elements/Series RLC Branch  PhysicalDomain=powersysdomain  SubClassName=unknown  LeftPortType=p1  RightPortType=p1  LConnTagsString=__new0  RConnTagsString=__new0  Resistance=6800  Inductance=0  Capacitance=inf  Measurements=None
  R2 : powerlib/Elements/Series RLC Branch  Orientation=up  PhysicalDomain=powersysdomain  SubClassName=unknown  LeftPortType=p1  RightPortType=p1  LConnTagsString=__new0  RConnTagsString=__new0  Resistance=4700  Inductance=0  Capacitance=inf  Measurements=None
  measure1 : powerlib/Measurements/Voltage Measurement  PhasorSimulation=off  OutputType=Magnitude  PSBequivalent=0
  output Ground2 : powerlib/Elements/Ground  Orientation=down  PhysicalDomain=powersysdomain  SubClassName=unknown  LeftPortType=p1  RightPortType=p1  LConnTagsString=a
  output Ground3 : powerlib/Elements/Ground  Orientation=down  PhysicalDomain=powersysdomain  SubClassName=unknown  LeftPortType=p1  RightPortType=p1  LConnTagsString=a
  Vin : PMIOPort  Port=1  Side=Left
  active : Outport
  wires:
  measure1/1 -> active/1
  connections:
  output Ground3/LConn1 -- measure1/LConn2
  output Ground2/LConn1 -- R2/LConn1
  Vin/RConn1 -- R1/LConn1
  measure1/LConn1 -- R2/RConn1 -- R1/RConn1

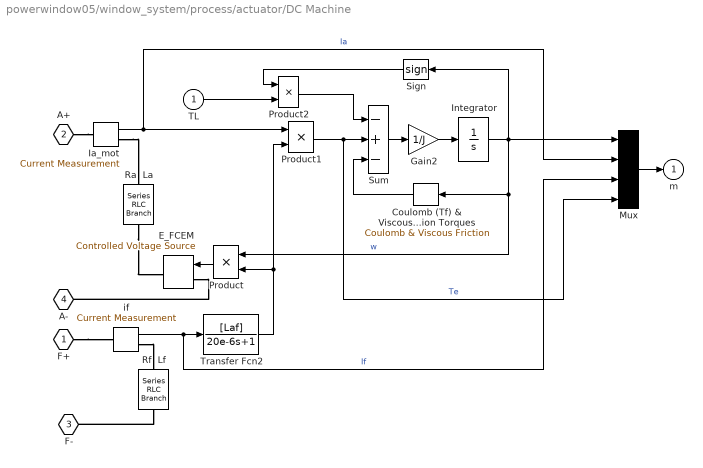
== system powerwindow05/window_system/process/actuator/DC Machine ==
  TL : Inport  Port=1  LatchInput=off
  Coulomb (Tf) & Viscous ( Bm*w)  Friction Torques : simulink/Discontinuities/Coulomb & Viscous Friction  Orientation=left  offset=Tf  gain=Bm
  E_FCEM : powerlib/Electrical Sources/Controlled Voltage Source  Orientation=left  Initialize=on  Amplitude=0  Phase=0  Frequency=0  Measurements=None
  Gain2 : Gain  Gain=1/J  SaturateOnIntegerOverflow=on
  Ia_mot : powerlib/Measurements/Current Measurement  PhasorSimulation=off  OutputType=Magnitude  PSBequivalent=0
  Integrator : Integrator  InitialCondition=w0
  Mux : Mux
  Product : Product  Orientation=left  SaturateOnIntegerOverflow=on  InputSameDT=on
  Product1 : Product  SaturateOnIntegerOverflow=on  InputSameDT=on
  Product2 : Product  SaturateOnIntegerOverflow=on  InputSameDT=on
  Ra  La : powerlib/Elements/Series RLC Branch  Orientation=down  PhysicalDomain=powersysdomain  SubClassName=unknown  LeftPortType=p1  RightPortType=p1  LConnTagsString=__new0  RConnTagsString=__new0  Resistance=Ra  Inductance=La  Capacitance=inf  Measurements=None
  Rf  Lf : powerlib/Elements/Series RLC Branch  Orientation=down  PhysicalDomain=powersysdomain  SubClassName=unknown  LeftPortType=p1  RightPortType=p1  LConnTagsString=__new0  RConnTagsString=__new0  Resistance=Rf  Inductance=Lf  Capacitance=inf  Measurements=None
  Sign : Signum  Orientation=left
  Sum : Sum  Inputs=-+-  SaturateOnIntegerOverflow=on  InputSameDT=on
  Transfer Fcn2 : TransferFcn  Numerator=[Laf]  Denominator=[20e-6 1]
  if : powerlib/Measurements/Current Measurement  PhasorSimulation=off  OutputType=Magnitude  PSBequivalent=0
  F+ : PMIOPort  Port=1  Side=Left
  A+ : PMIOPort  Port=2  Side=Left
  F- : PMIOPort  Port=3  Side=Right
  A- : PMIOPort  Port=4  Side=Right
  m : Outport  InitialOutput=0
  wires:
  Ia_mot/1 -> Product1/1, Mux/2  "Ia"
  if/1 -> Transfer Fcn2/1, Mux/3  "If"
  Product/1 -> E_FCEM/1
  Product2/1 -> Sum/1
  TL/1 -> Product2/2
  Sign/1 -> Product2/1
  Sum/1 -> Gain2/1
  Gain2/1 -> Integrator/1
  Integrator/1 -> Coulomb (Tf) & Viscous ( Bm*w)  Friction Torques/1, Product/1, Mux/1, Sign/1  "w"
  Product1/1 -> Sum/2, Mux/4  "Te"
  Mux/1 -> m/1
  Transfer Fcn2/1 -> Product1/2, Product/2
  Coulomb (Tf) & Viscous ( Bm*w)  Friction Torques/1 -> Sum/3
  connections:
  Ra  La/RConn1 -- E_FCEM/RConn1
  A+/RConn1 -- Ia_mot/LConn1
  Ia_mot/RConn1 -- Ra  La/LConn1
  F+/RConn1 -- if/LConn1
  if/RConn1 -- Rf  Lf/LConn1
  E_FCEM/LConn1 -- A-/RConn1
  Rf  Lf/RConn1 -- F-/RConn1

== system powerwindow05/window_system/process/actuator/Demux ==
  m : Inport  Port=1  LatchInput=off
  Demux : Demux
  wm : Outport
  Ia : Outport  Port=2
  If : Outport  Port=3
  Te : Outport  Port=4
  wires:
  Demux/1 -> wm/1
  Demux/2 -> Ia/1
  m/1 -> Demux/1
  Demux/3 -> If/1
  Demux/4 -> Te/1

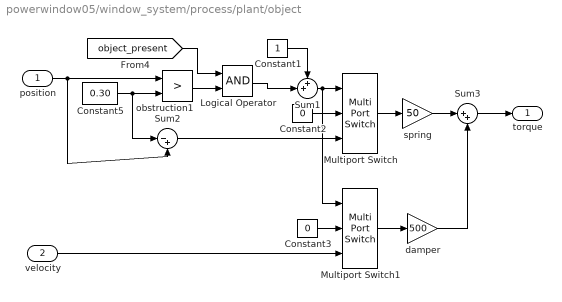
== system powerwindow05/window_system/process/plant/object ==
  position : Inport  Port=1  LatchInput=off
  velocity : Inport  Port=2  LatchInput=off
  Constant1 : Constant
  Constant2 : Constant  Value=0
  Constant3 : Constant  Value=0
  Constant5 : Constant  Value=0.30
  Logical Operator : Logic
  Multiport Switch : MultiPortSwitch  Inputs=2  InputSameDT=on
  Multiport Switch1 : MultiPortSwitch  Inputs=2  InputSameDT=on
  Sum1 : Sum  Inputs=++|  SaturateOnIntegerOverflow=on  InputSameDT=on
  Sum2 : Sum  Inputs=|-+  SaturateOnIntegerOverflow=on  InputSameDT=on
  Sum3 : Sum  Inputs=|++  SaturateOnIntegerOverflow=on  InputSameDT=on
  damper : Gain  Gain=500  SaturateOnIntegerOverflow=on
  obstruction1 : RelationalOperator  Operator=>  InputSameDT=on
  spring : Gain  Gain=50  SaturateOnIntegerOverflow=on
  torque : Outport
  wires:
  [object_present] -> Logical Operator/1
  Logical Operator/1 -> Sum1/2
  obstruction1/1 -> Logical Operator/2
  Multiport Switch1/1 -> damper/1
  velocity/1 -> Multiport Switch1/3
  Constant3/1 -> Multiport Switch1/2
  Multiport Switch/1 -> spring/1
  position/1 -> Sum2/2, obstruction1/1
  Constant1/1 -> Sum1/1
  Sum2/1 -> Multiport Switch/3
  Constant2/1 -> Multiport Switch/2
  Sum1/1 -> Multiport Switch1/1, Multiport Switch/1
  Constant5/1 -> Sum2/1, obstruction1/2
  damper/1 -> Sum3/2
  Sum3/1 -> torque/1
  spring/1 -> Sum3/1
